simulink model "Prismatic_Power_Simulink"  (R2021a)
settings: Solver=VariableStepAuto  StartTime=0.0  StopTime=10.0  RelTol=1e-3
libraries: fl_lib x62, nesl_utility x24, fl_ps_legacy_lib x16, ee_lib x7, pid_lib x3, simulink x2
(part 2 of 2)

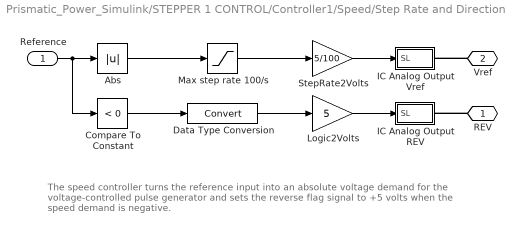
== system Prismatic_Power_Simulink/STEPPER 1 CONTROL/Controller1/Speed/Step Rate and Direction ==
  note: The speed controller turns the reference input into an absolute voltage demand for the
      | voltage-controlled pulse generator and sets the reverse flag signal to +5 volts when the
      | speed demand is negative.
  Reference : Inport  RequirementInfo={} %GIDa_ffddedba_40a7_4d42_9e04_5d0d4bf26553
  Abs : Abs  RequirementInfo={} %GIDa_dea4ee78_c76c_47ee_8a07_a6520ce0509a
  Compare To Constant : simulink/Logic and Bit Operations/Compare To Constant  RequirementInfo={} %GIDa_1e0f1a2a_a61c_4b0a_b1de_cea5422492ce  relop=<  const=0  OutDataTypeStr=uint8  ZeroCross=off
  Data Type Conversion : DataTypeConversion  RequirementInfo={} %GIDa_f4275750_c3e2_45d8_b8eb_9180457155cd
  IC Analog Output REV : Subsystem  RequirementInfo={} %GIDa_7f0cb09f_9968_43ae_a898_3e557d5eb4b3
  IC Analog Output Vref : Subsystem  RequirementInfo={} %GIDa_89d529e8_f418_4cf0_bc64_5937d193629e
  Logic2Volts : Gain  RequirementInfo={} %GIDa_00a6a936_49a5_4604_ae7a_8331545a55e7  Gain=5
  Max step rate 100/s : Saturate  RequirementInfo={} %GIDa_59a219ac_010f_49ac_9c05_5584bb84e902  UpperLimit=100  LowerLimit=0
  StepRate2Volts : Gain  RequirementInfo={} %GIDa_49ff8043_9ae2_4473_be11_4e49db1e5955  Gain=5/100
  REV : PMIOPort  RequirementInfo={} %GIDa_48fb72ab_978f_4af6_96a9_fcbf31071fb3  Side=Right
  Vref : PMIOPort  RequirementInfo={} %GIDa_b9e70f5d_42a5_47c9_b646_40bbfda27cae  Port=2  Side=Right
  wires:
  StepRate2Volts/1 -> IC Analog Output Vref/1(SL)
  Max step rate 100/s/1 -> StepRate2Volts/1
  Data Type Conversion/1 -> Logic2Volts/1
  Compare To Constant/1 -> Data Type Conversion/1
  Reference/1 -> Compare To Constant/1, Abs/1
  Abs/1 -> Max step rate 100/s/1
  Logic2Volts/1 -> IC Analog Output REV/1(SL)
  connections:
  REV/RConn1 -- IC Analog Output REV/RConn1
  Vref/RConn1 -- IC Analog Output Vref/RConn1

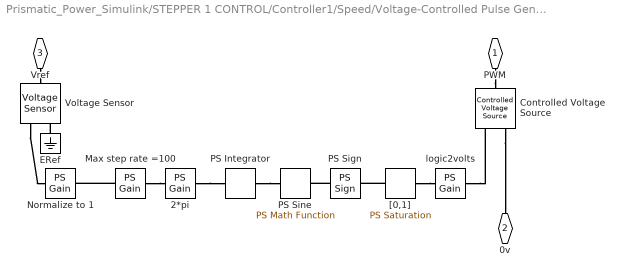
== system Prismatic_Power_Simulink/STEPPER 1 CONTROL/Controller1/Speed/Voltage-Controlled Pulse Generator ==
  2*pi : fl_ps_legacy_lib/Legacy Physical Signals/Functions/PS Gain  RequirementInfo={} %GIDa_bb742e79_5fd4_4dde_936d_5693eceb73d2  gain=-2*pi
  Controlled Voltage Source : fl_lib/Electrical/Electrical Sources/Controlled Voltage Source  RequirementInfo={} %GIDa_d6213159_ac1a_43a7_b50a_81c450da817d
  ERef : fl_lib/Electrical/Electrical Elements/Electrical Reference  RequirementInfo={} %GIDa_474626e3_68f1_4209_b449_fb4d8060caae
  Max step rate =100 : fl_ps_legacy_lib/Legacy Physical Signals/Functions/PS Gain  RequirementInfo={} %GIDa_0c8da716_440e_4856_b87d_ace4d9d5b5b3  gain=100
  Normalize to 1 : fl_ps_legacy_lib/Legacy Physical Signals/Functions/PS Gain  RequirementInfo={} %GIDa_b7843a87_27db_4020_9424_e6284065d874  gain=1/5
  PS Integrator : fl_ps_legacy_lib/Legacy Physical Signals/Linear Operators/PS Integrator  RequirementInfo={} %GIDa_64e510bc_2b7e_4553_a299_aafe5e399715  x0=0
      settings: SourceProductBaseCode=SS  InternalSimscapePortConfiguration="{\"Bottom\":[],\"Left\":[{\"id\":\"I\",\"label\":\"\",\"type\":\"input\"}],\"Right\":[{\"id\":\"O\",\"label\":\"\",\"type\":\"output\"}],\"Top\":[]}"
  PS Sign : fl_ps_legacy_lib/Legacy Physical Signals/Nonlinear Operators/PS Sign  RequirementInfo={} %GIDa_c00c01c9_5df2_4f73_b563_17c1cd493c8c
      settings: SourceProductBaseCode=SS  InternalSimscapePortConfiguration="{\"Bottom\":[],\"Left\":[{\"id\":\"I\",\"label\":\"\",\"type\":\"input\"}],\"Right\":[{\"id\":\"O\",\"label\":\"\",\"type\":\"output\"}],\"Top\":[]}"
  PS Sine : fl_ps_legacy_lib/Legacy Physical Signals/Functions/PS Math Function  RequirementInfo={} %GIDa_910a32a0_f1e5_427c_9126_70830ba9a458  fcn_choice=1
      settings: SourceProductBaseCode=SS  InternalSimscapePortConfiguration="{\"Bottom\":[],\"Left\":[{\"id\":\"I\",\"label\":\"\",\"type\":\"input\"}],\"Right\":[{\"id\":\"O\",\"label\":\"\",\"type\":\"output\"}],\"Top\":[]}"
  Voltage Sensor : fl_lib/Electrical/Electrical Sensors/Voltage Sensor  RequirementInfo={} %GIDa_f19b1ffe_bbee_469c_892a_953ea4e5dc3d
  "[0,1]" : fl_ps_legacy_lib/Legacy Physical Signals/Nonlinear Operators/PS Saturation  RequirementInfo={} %GIDa_60b1a7bc_aa18_42d8_8ef2_6fff1dadf3d3  upper_limit=1  lower_limit=0
      settings: SourceProductBaseCode=SS  InternalSimscapePortConfiguration="{\"Bottom\":[],\"Left\":[{\"id\":\"I\",\"label\":\"\",\"type\":\"input\"}],\"Right\":[{\"id\":\"O\",\"label\":\"\",\"type\":\"output\"}],\"Top\":[]}"
  logic2volts : fl_ps_legacy_lib/Legacy Physical Signals/Functions/PS Gain  RequirementInfo={} %GIDa_b55addc7_ecd5_44cf_abb7_b23590426edd  gain=5
  PWM : PMIOPort  RequirementInfo={} %GIDa_326e9d1b_9187_41a9_99ea_c7a847ec9af9  Side=Right
  0v : PMIOPort  RequirementInfo={} %GIDa_96144acc_2519_4ff7_8196_dca1dedb656a  Port=2  Side=Right
  Vref : PMIOPort  RequirementInfo={} %GIDa_12d0c042_a145_4fe4_a178_7cc42b57f5cf  Port=3  Side=Left
  connections:
  PWM/RConn1 -- Controlled Voltage Source/LConn1
  Controlled Voltage Source/RConn2 -- 0v/RConn1
  Vref/RConn1 -- Voltage Sensor/LConn1
  ERef/LConn1 -- Voltage Sensor/RConn2
  Voltage Sensor/RConn1 -- Normalize to 1/LConn1
  Max step rate =100/LConn1 -- Normalize to 1/RConn1
  Max step rate =100/RConn1 -- 2*pi/LConn1
  2*pi/RConn1 -- PS Integrator/LConn1
  PS Integrator/RConn1 -- PS Sine/LConn1
  PS Sign/LConn1 -- PS Sine/RConn1
  "[0,1]"/LConn1 -- PS Sign/RConn1
  "[0,1]"/RConn1 -- logic2volts/LConn1
  logic2volts/RConn1 -- Controlled Voltage Source/RConn1

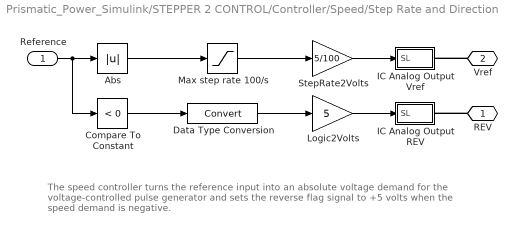
== system Prismatic_Power_Simulink/STEPPER 2 CONTROL/Controller/Speed/Step Rate and Direction ==
  note: The speed controller turns the reference input into an absolute voltage demand for the
      | voltage-controlled pulse generator and sets the reverse flag signal to +5 volts when the
      | speed demand is negative.
  Reference : Inport  RequirementInfo={} %GIDa_f0f74585_f7e1_4bc2_a7b8_7fbae9e2ef1e
  Abs : Abs  RequirementInfo={} %GIDa_9919b9a9_868b_44ea_979d_73c2b80415d3
  Compare To Constant : simulink/Logic and Bit Operations/Compare To Constant  RequirementInfo={} %GIDa_9fb11882_0a12_42b5_9b25_c521b0743134  relop=<  const=0  OutDataTypeStr=uint8  ZeroCross=off
  Data Type Conversion : DataTypeConversion  RequirementInfo={} %GIDa_d2ef139c_ee5e_4b26_8a93_23f86a4d4d82
  IC Analog Output REV : Subsystem  RequirementInfo={} %GIDa_10774651_ac5e_4b06_bdfd_9cadd4e79075
  IC Analog Output Vref : Subsystem  RequirementInfo={} %GIDa_ae56f616_b3c6_4bed_9094_c5738d3f86ca
  Logic2Volts : Gain  RequirementInfo={} %GIDa_c833c559_5c5a_4bf7_924b_94d681a31fbb  Gain=5
  Max step rate 100/s : Saturate  RequirementInfo={} %GIDa_3b859d89_f371_464f_9686_dc502b35f252  UpperLimit=100  LowerLimit=0
  StepRate2Volts : Gain  RequirementInfo={} %GIDa_fd19fb8a_875e_4627_b2a5_5c3814a10b3d  Gain=5/100
  REV : PMIOPort  RequirementInfo={} %GIDa_6ec3933a_6f5a_48b2_a9d3_d0b70d726a5c  Side=Right
  Vref : PMIOPort  RequirementInfo={} %GIDa_a6bc400b_17be_4c93_a815_e7608ab59bfd  Port=2  Side=Right
  wires:
  StepRate2Volts/1 -> IC Analog Output Vref/1(SL)
  Max step rate 100/s/1 -> StepRate2Volts/1
  Data Type Conversion/1 -> Logic2Volts/1
  Compare To Constant/1 -> Data Type Conversion/1
  Reference/1 -> Compare To Constant/1, Abs/1
  Abs/1 -> Max step rate 100/s/1
  Logic2Volts/1 -> IC Analog Output REV/1(SL)
  connections:
  REV/RConn1 -- IC Analog Output REV/RConn1
  Vref/RConn1 -- IC Analog Output Vref/RConn1

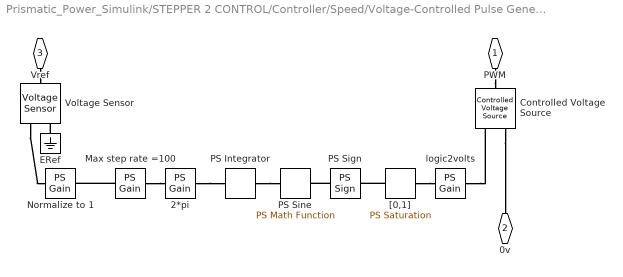
== system Prismatic_Power_Simulink/STEPPER 2 CONTROL/Controller/Speed/Voltage-Controlled Pulse Generator ==
  2*pi : fl_ps_legacy_lib/Legacy Physical Signals/Functions/PS Gain  RequirementInfo={} %GIDa_d62d9fb4_6538_4c68_9991_8cd57bd9b074  gain=-2*pi
  Controlled Voltage Source : fl_lib/Electrical/Electrical Sources/Controlled Voltage Source  RequirementInfo={} %GIDa_212d009f_269b_4782_a86d_0855625fe586
  ERef : fl_lib/Electrical/Electrical Elements/Electrical Reference  RequirementInfo={} %GIDa_fec843c6_b520_4239_b220_1d02ee843d19
  Max step rate =100 : fl_ps_legacy_lib/Legacy Physical Signals/Functions/PS Gain  RequirementInfo={} %GIDa_b65954cb_feb8_4e59_add4_87f15724c57f  gain=100
  Normalize to 1 : fl_ps_legacy_lib/Legacy Physical Signals/Functions/PS Gain  RequirementInfo={} %GIDa_da0e996b_c324_4bcc_a864_28c814484b5e  gain=1/5
  PS Integrator : fl_ps_legacy_lib/Legacy Physical Signals/Linear Operators/PS Integrator  RequirementInfo={} %GIDa_2d1bda21_ef73_4afa_8cf9_867110f7619c  x0=0
      settings: SourceProductBaseCode=SS  InternalSimscapePortConfiguration="{\"Bottom\":[],\"Left\":[{\"id\":\"I\",\"label\":\"\",\"type\":\"input\"}],\"Right\":[{\"id\":\"O\",\"label\":\"\",\"type\":\"output\"}],\"Top\":[]}"
  PS Sign : fl_ps_legacy_lib/Legacy Physical Signals/Nonlinear Operators/PS Sign  RequirementInfo={} %GIDa_f571f63c_d450_4422_bacb_a50f5ccf8185
      settings: SourceProductBaseCode=SS  InternalSimscapePortConfiguration="{\"Bottom\":[],\"Left\":[{\"id\":\"I\",\"label\":\"\",\"type\":\"input\"}],\"Right\":[{\"id\":\"O\",\"label\":\"\",\"type\":\"output\"}],\"Top\":[]}"
  PS Sine : fl_ps_legacy_lib/Legacy Physical Signals/Functions/PS Math Function  RequirementInfo={} %GIDa_d7cf9ef2_6e59_4c9c_86db_c6bd6ef512f4  fcn_choice=1
      settings: SourceProductBaseCode=SS  InternalSimscapePortConfiguration="{\"Bottom\":[],\"Left\":[{\"id\":\"I\",\"label\":\"\",\"type\":\"input\"}],\"Right\":[{\"id\":\"O\",\"label\":\"\",\"type\":\"output\"}],\"Top\":[]}"
  Voltage Sensor : fl_lib/Electrical/Electrical Sensors/Voltage Sensor  RequirementInfo={} %GIDa_e45057a7_50d7_4fe5_9e1a_d86eb06f0ccb
  "[0,1]" : fl_ps_legacy_lib/Legacy Physical Signals/Nonlinear Operators/PS Saturation  RequirementInfo={} %GIDa_5404380f_b4f2_4da5_8991_341a42738530  upper_limit=1  lower_limit=0
      settings: SourceProductBaseCode=SS  InternalSimscapePortConfiguration="{\"Bottom\":[],\"Left\":[{\"id\":\"I\",\"label\":\"\",\"type\":\"input\"}],\"Right\":[{\"id\":\"O\",\"label\":\"\",\"type\":\"output\"}],\"Top\":[]}"
  logic2volts : fl_ps_legacy_lib/Legacy Physical Signals/Functions/PS Gain  RequirementInfo={} %GIDa_edd6e3dd_c58e_4c3c_aece_c640391a8f36  gain=5
  PWM : PMIOPort  RequirementInfo={} %GIDa_1bb188b6_b97d_46b1_a11f_7366021f3e37  Side=Right
  0v : PMIOPort  RequirementInfo={} %GIDa_088bcef0_c308_4f54_8adb_c12c2a75574d  Port=2  Side=Right
  Vref : PMIOPort  RequirementInfo={} %GIDa_fea449ad_d460_431e_9c72_9db32530dfd8  Port=3  Side=Left
  connections:
  PWM/RConn1 -- Controlled Voltage Source/LConn1
  Controlled Voltage Source/RConn2 -- 0v/RConn1
  Vref/RConn1 -- Voltage Sensor/LConn1
  ERef/LConn1 -- Voltage Sensor/RConn2
  Voltage Sensor/RConn1 -- Normalize to 1/LConn1
  Max step rate =100/LConn1 -- Normalize to 1/RConn1
  Max step rate =100/RConn1 -- 2*pi/LConn1
  2*pi/RConn1 -- PS Integrator/LConn1
  PS Integrator/RConn1 -- PS Sine/LConn1
  PS Sign/LConn1 -- PS Sine/RConn1
  "[0,1]"/LConn1 -- PS Sign/RConn1
  "[0,1]"/RConn1 -- logic2volts/LConn1
  logic2volts/RConn1 -- Controlled Voltage Source/RConn1

== system Prismatic_Power_Simulink/STEPPER 1 CONTROL/Controller1/Position/Algorithm and Pulse Generation/IC Analog Output REV ==
  SL : Inport  RequirementInfo={} %GIDa_b96a42a5_075b_418b_aa97_43b85aba5bc8
  Controlled Voltage Source : fl_lib/Electrical/Electrical Sources/Controlled Voltage Source  RequirementInfo={} %GIDa_d56cc304_62d2_4b19_b0d8_fcde141a5274
  ERef : fl_lib/Electrical/Electrical Elements/Electrical Reference  RequirementInfo={} %GIDa_efad5ee6_896e_4160_9e99_1adcceac10da
  Simulink-PS Converter : nesl_utility/Simulink-PS Converter  RequirementInfo={} %GIDa_d2c5c693_f6cf_4267_a2f9_389637385eee  PhysicalDomain=network_engine_domain  SubClassName=ps_input  LeftPortType=input  RightPortType=output  PseudoPeriodic=off  Frequencies=[]  NoiseDistribution=none  NoiseParameters=[]  Unit=V  AffineConversion=off  FilteringAndDerivatives=zero  SimscapeFilterOrder=1  InputFilterTimeConstant=.001  UdotUserProvided=0
      settings: SourceProductBaseCode=PW,SS
  V : PMIOPort  RequirementInfo={} %GIDa_13a759cc_60c8_4408_be71_2238b5acc643  Side=Right
  wires:
  SL/1 -> Simulink-PS Converter/1
  connections:
  ERef/LConn1 -- Controlled Voltage Source/RConn2
  V/RConn1 -- Controlled Voltage Source/LConn1
  Simulink-PS Converter/RConn1 -- Controlled Voltage Source/RConn1

== system Prismatic_Power_Simulink/STEPPER 1 CONTROL/Controller1/Position/Algorithm and Pulse Generation/IC Analog Output Vref ==
  SL : Inport  RequirementInfo={} %GIDa_cce4ebc6_f53c_441e_83f9_2cb4e097bd83
  Controlled Voltage Source : fl_lib/Electrical/Electrical Sources/Controlled Voltage Source  RequirementInfo={} %GIDa_d25fee1c_c1cb_4341_980f_7b059d3b9a56
  ERef : fl_lib/Electrical/Electrical Elements/Electrical Reference  RequirementInfo={} %GIDa_e837ef32_9930_4a44_8eba_e986dfa546a7
  Simulink-PS Converter : nesl_utility/Simulink-PS Converter  RequirementInfo={} %GIDa_3992de25_48cf_4a4b_a2f0_5f14a93708be  PhysicalDomain=network_engine_domain  SubClassName=ps_input  LeftPortType=input  RightPortType=output  PseudoPeriodic=off  Frequencies=[]  NoiseDistribution=none  NoiseParameters=[]  Unit=V  AffineConversion=off  FilteringAndDerivatives=zero  SimscapeFilterOrder=1  InputFilterTimeConstant=.001  UdotUserProvided=0
      settings: SourceProductBaseCode=PW,SS
  V : PMIOPort  RequirementInfo={} %GIDa_d3cf80a6_7c78_4a45_9047_f86f131b5967  Side=Right
  wires:
  SL/1 -> Simulink-PS Converter/1
  connections:
  Simulink-PS Converter/RConn1 -- Controlled Voltage Source/RConn1
  V/RConn1 -- Controlled Voltage Source/LConn1
  ERef/LConn1 -- Controlled Voltage Source/RConn2

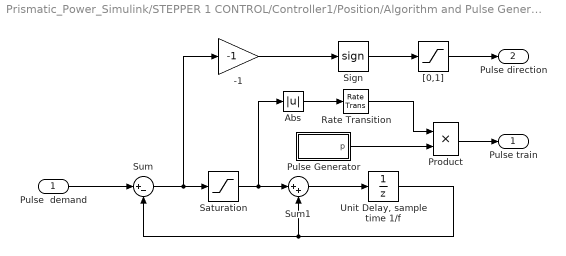
== system Prismatic_Power_Simulink/STEPPER 1 CONTROL/Controller1/Position/Algorithm and Pulse Generation/Pulse Generator ==
  Pulse  demand : Inport  RequirementInfo={} %GIDa_431bed87_e9e6_4858_8e8f_f4453a5c4a0f  SampleTime=1/f
  -1 : Gain  RequirementInfo={} %GIDa_f6c93b2d_9163_42d2_96f3_45ee38615d73  Gain=-1
  Abs : Abs  RequirementInfo={} %GIDa_ccd32744_4105_423d_add9_ca93638f073b
  Product : Product  RequirementInfo={} %GIDa_f347e8b5_91fb_4d17_b6ad_da1bfbcd38cc  InputSameDT=on  SaturateOnIntegerOverflow=on  OutDataTypeStr=Inherit: Same as first input
  Pulse Generator : Subsystem  RequirementInfo={} %GIDa_0ec43f8b_06e6_472c_b565_421411fb8ee7
  Rate Transition : RateTransition  RequirementInfo={} %GIDa_63e9a268_7461_450e_8dd7_75865fbb0ef3  Deterministic=off
  Saturation : Saturate  RequirementInfo={} %GIDa_00f825ab_0dfa_446b_860b_0eb8a6f4521d  UpperLimit=1  LowerLimit=-1
  Sign : Signum  RequirementInfo={} %GIDa_c30efebc_e2d0_41f8_b87d_2ae7576419ef
  Sum : Sum  RequirementInfo={} %GIDa_6cb3f66b_c50e_472e_aa2d_aa688b39c928  Inputs=|+-
  Sum1 : Sum  RequirementInfo={} %GIDa_cc032205_ac52_4a30_ba23_fe89b77453b9  Inputs=|++
  "Unit Delay, sample time 1/f" : UnitDelay  RequirementInfo={} %GIDa_490fa863_23ab_42f1_b08e_0683f2637e70  SampleTime=1/f  HasFrameUpgradeWarning=on
  "[0,1]" : Saturate  RequirementInfo={} %GIDa_5ff7bd16_081b_4eb2_9313_4cd2024583c7  UpperLimit=1  LowerLimit=0
  Pulse train : Outport  RequirementInfo={} %GIDa_6d098edf_a3e3_4fdc_9240_6302a77a0a00  VectorParamsAs1DForOutWhenUnconnected=off
  Pulse direction : Outport  RequirementInfo={} %GIDa_d7ef0ffd_0ca5_4aff_bcae_597eee077a4b  Port=2  VectorParamsAs1DForOutWhenUnconnected=off
  wires:
  "[0,1]"/1 -> Pulse direction/1
  -1/1 -> Sign/1
  "Unit Delay, sample time 1/f"/1 -> Sum/2, Sum1/2
  Pulse  demand/1 -> Sum/1
  Sum/1 -> -1/1, Saturation/1
  Saturation/1 -> Sum1/1, Abs/1
  Sum1/1 -> "Unit Delay, sample time 1/f"/1
  Sign/1 -> "[0,1]"/1
  Product/1 -> Pulse train/1
  Abs/1 -> Rate Transition/1
  Pulse Generator/1(p) -> Product/2
  Rate Transition/1 -> Product/1

== system Prismatic_Power_Simulink/STEPPER 1 CONTROL/Controller1/Speed/Step Rate and Direction/IC Analog Output REV ==
  SL : Inport  RequirementInfo={} %GIDa_d57de94e_c6c0_4888_8674_d8add924f614
  Controlled Voltage Source : fl_lib/Electrical/Electrical Sources/Controlled Voltage Source  RequirementInfo={} %GIDa_0688e754_8ea5_4a3d_a2d2_35a2d1ca19b3
  ERef : fl_lib/Electrical/Electrical Elements/Electrical Reference  RequirementInfo={} %GIDa_7625d271_bfb6_4a5b_943e_51dae823b210
  Simulink-PS Converter : nesl_utility/Simulink-PS Converter  RequirementInfo={} %GIDa_6440d5f0_dda0_49df_b14d_1fd16b902c8a  PhysicalDomain=network_engine_domain  SubClassName=ps_input  LeftPortType=input  RightPortType=output  PseudoPeriodic=off  Frequencies=[]  NoiseDistribution=none  NoiseParameters=[]  Unit=V  AffineConversion=off  FilteringAndDerivatives=zero  SimscapeFilterOrder=1  InputFilterTimeConstant=.001  UdotUserProvided=0
      settings: SourceProductBaseCode=PW,SS
  V : PMIOPort  RequirementInfo={} %GIDa_932a4365_b524_4758_9264_02d920f21d64  Side=Right
  wires:
  SL/1 -> Simulink-PS Converter/1
  connections:
  Simulink-PS Converter/RConn1 -- Controlled Voltage Source/RConn1
  V/RConn1 -- Controlled Voltage Source/LConn1
  ERef/LConn1 -- Controlled Voltage Source/RConn2

== system Prismatic_Power_Simulink/STEPPER 1 CONTROL/Controller1/Speed/Step Rate and Direction/IC Analog Output Vref ==
  SL : Inport  RequirementInfo={} %GIDa_f561b98b_70b1_43f6_bb3d_87e36387313c
  Controlled Voltage Source : fl_lib/Electrical/Electrical Sources/Controlled Voltage Source  RequirementInfo={} %GIDa_937b1feb_0a53_482b_a2ad_b99dd2b4dd90
  ERef : fl_lib/Electrical/Electrical Elements/Electrical Reference  RequirementInfo={} %GIDa_898e64a2_d6a0_4dc8_b8f8_0e1845fdb571
  Simulink-PS Converter : nesl_utility/Simulink-PS Converter  RequirementInfo={} %GIDa_5430a408_fdc5_4d93_ac8e_88d347a8322b  PhysicalDomain=network_engine_domain  SubClassName=ps_input  LeftPortType=input  RightPortType=output  PseudoPeriodic=off  Frequencies=[]  NoiseDistribution=none  NoiseParameters=[]  Unit=V  AffineConversion=off  FilteringAndDerivatives=zero  SimscapeFilterOrder=1  InputFilterTimeConstant=.001  UdotUserProvided=0
      settings: SourceProductBaseCode=PW,SS
  V : PMIOPort  RequirementInfo={} %GIDa_d53b4e64_9f3c_4e8e_8a43_47300ce19d48  Side=Right
  wires:
  SL/1 -> Simulink-PS Converter/1
  connections:
  ERef/LConn1 -- Controlled Voltage Source/RConn2
  V/RConn1 -- Controlled Voltage Source/LConn1
  Simulink-PS Converter/RConn1 -- Controlled Voltage Source/RConn1

== system Prismatic_Power_Simulink/STEPPER 2 CONTROL/Controller/Speed/Step Rate and Direction/IC Analog Output REV ==
  SL : Inport  RequirementInfo={} %GIDa_7b13e009_a7b4_4e47_a0cf_01527f25aed0
  Controlled Voltage Source : fl_lib/Electrical/Electrical Sources/Controlled Voltage Source  RequirementInfo={} %GIDa_00a9daab_5825_448d_97b4_efeebb9eec76
  ERef : fl_lib/Electrical/Electrical Elements/Electrical Reference  RequirementInfo={} %GIDa_80fa04fd_4341_4024_960c_84f7416955ee
  Simulink-PS Converter : nesl_utility/Simulink-PS Converter  RequirementInfo={} %GIDa_1fbeb92e_4e2b_48a7_9610_770646752645  PhysicalDomain=network_engine_domain  SubClassName=ps_input  LeftPortType=input  RightPortType=output  PseudoPeriodic=off  Frequencies=[]  NoiseDistribution=none  NoiseParameters=[]  Unit=V  AffineConversion=off  FilteringAndDerivatives=zero  SimscapeFilterOrder=1  InputFilterTimeConstant=.001  UdotUserProvided=0
      settings: SourceProductBaseCode=PW,SS
  V : PMIOPort  RequirementInfo={} %GIDa_da1122a8_59a1_43ca_8758_a182ba3d3f6e  Side=Right
  wires:
  SL/1 -> Simulink-PS Converter/1
  connections:
  Simulink-PS Converter/RConn1 -- Controlled Voltage Source/RConn1
  V/RConn1 -- Controlled Voltage Source/LConn1
  ERef/LConn1 -- Controlled Voltage Source/RConn2

== system Prismatic_Power_Simulink/STEPPER 2 CONTROL/Controller/Speed/Step Rate and Direction/IC Analog Output Vref ==
  SL : Inport  RequirementInfo={} %GIDa_7300c9d3_4c8d_4720_94cc_0a4cf1ad7f69
  Controlled Voltage Source : fl_lib/Electrical/Electrical Sources/Controlled Voltage Source  RequirementInfo={} %GIDa_10c77bfe_3884_4f38_a082_58d8e7ef0ecd
  ERef : fl_lib/Electrical/Electrical Elements/Electrical Reference  RequirementInfo={} %GIDa_2b8fa4ac_e18f_4763_84d8_4207fa9d0053
  Simulink-PS Converter : nesl_utility/Simulink-PS Converter  RequirementInfo={} %GIDa_5abdd284_25be_4d0c_8651_738aff1ad7a3  PhysicalDomain=network_engine_domain  SubClassName=ps_input  LeftPortType=input  RightPortType=output  PseudoPeriodic=off  Frequencies=[]  NoiseDistribution=none  NoiseParameters=[]  Unit=V  AffineConversion=off  FilteringAndDerivatives=zero  SimscapeFilterOrder=1  InputFilterTimeConstant=.001  UdotUserProvided=0
      settings: SourceProductBaseCode=PW,SS
  V : PMIOPort  RequirementInfo={} %GIDa_129f666d_1816_48cd_80fe_21f733a79909  Side=Right
  wires:
  SL/1 -> Simulink-PS Converter/1
  connections:
  ERef/LConn1 -- Controlled Voltage Source/RConn2
  V/RConn1 -- Controlled Voltage Source/LConn1
  Simulink-PS Converter/RConn1 -- Controlled Voltage Source/RConn1

== system Prismatic_Power_Simulink/STEPPER 1 CONTROL/Controller1/Position/Algorithm and Pulse Generation/Pulse Generator/Pulse Generator ==
  -1 : Gain  RequirementInfo={} %GIDa_35f9443c_8d8e_40de_a8eb_aaa41cb8bdb3  Gain=0.5
  Constant : Constant  RequirementInfo={} %GIDa_10a13dd4_814b_4986_8d87_cf80efe3a36e  SampleTime=1/(2*f)
  Gain : Gain  RequirementInfo={} %GIDa_0550593f_0555_450a_9ebf_a8be59820d88  Gain=-1
  Sum : Sum  RequirementInfo={} %GIDa_7d504e48_3c8e_4fe9_b89d_78d220ac48a0  Inputs=|++
  "Unit Delay, sample time 1/2*f)" : UnitDelay  RequirementInfo={} %GIDa_487ffcb2_8a2f_4866_b442_d78a25438b66  InitialCondition=-1  SampleTime=1/(2*f)  HasFrameUpgradeWarning=on
  p : Outport  RequirementInfo={} %GIDa_17ce2762_66a9_48b2_abed_a999f38705ca  VectorParamsAs1DForOutWhenUnconnected=off
  wires:
  "Unit Delay, sample time 1/2*f)"/1 -> Gain/1, Sum/1
  Gain/1 -> "Unit Delay, sample time 1/2*f)"/1
  Constant/1 -> Sum/2
  Sum/1 -> -1/1
  -1/1 -> p/1

== matlab function Prismatic_Power_Simulink/Coordinate conversion ==
  data: x input; azimuth output; y input; z input; elevation output; r output
function [azimuth,elevation,r] = fcn(x, y, z)

    [azimuth,elevation,r] = cart2sph(x,y,z);
    azimuth = rad2deg(azimuth);
    elevation = rad2deg(elevation);

end
